simulink model "controller"  (R2024b)
settings: Solver=ode1  StartTime=0.0  StopTime=inf  FixedStep=0.01  RelTol=1e-3
libraries: robotlib x4, robotgazebolib x1
settings Model: Creator=abanesjo  LastModifiedBy=abanesjo

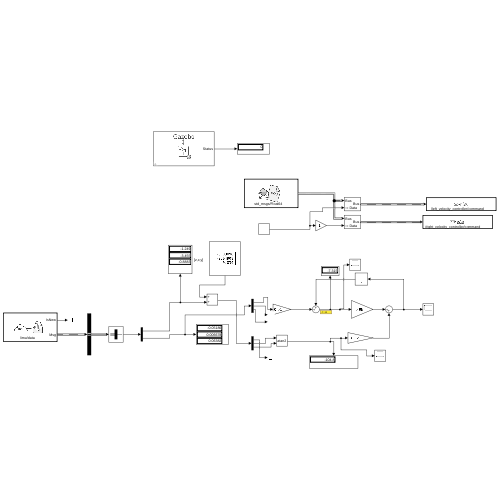
[thumbnail: Simulink's stored preview of the top-level diagram]
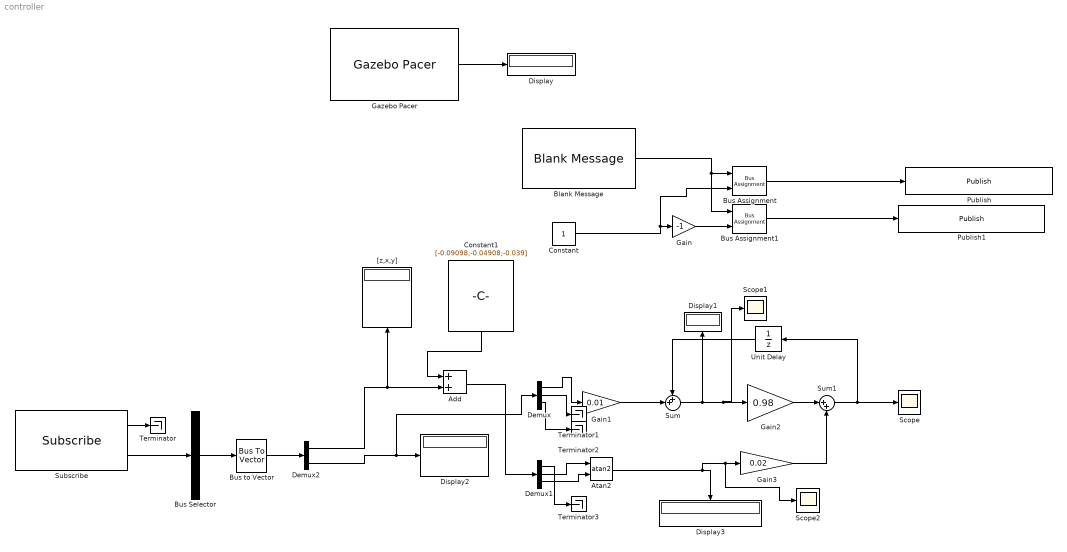
== system controller ==
  Add : Sum
  Atan2 : Trigonometry  Operator=atan2
  Blank Message : robotlib/Blank Message  messageClass=Message  entityType=std_msgs/Float64  messageType=std_msgs/Float64  SampleTime=inf  legacyBusStruct=off
  Bus Assignment : BusAssignment  AssignedSignals=Data
  Bus Assignment1 : BusAssignment  AssignedSignals=Data
  Bus Selector : BusSelector  OutputSignals=LinearAcceleration,AngularVelocity  OutputAsBus=on
  Bus to Vector : BusToVector
  Constant : Constant
  Constant1 : Constant  Value=[-0.09098;-0.04908;-0.039]  VectorParams1D=off
  Demux : Demux  Outputs=3
  Demux1 : Demux  Outputs=3
  Demux2 : Demux  Outputs=2
  Display{,1..3} (4 alike) : Display
  Gain : Gain  Gain=-1
  Gain1 : Gain  Gain=0.01
  Gain2 : Gain  Gain=0.98
  Gain3 : Gain  Gain=0.02
  Gazebo Pacer : robotgazebolib/Gazebo Pacer  ResetBehavior=Reset Gazebo simulation time and scene  SampleTime=0.01
  Publish : robotlib/Publish  topicSource=Specify your own  topic=/left_velocity_controller/command  messageType=std_msgs/Float64  legacyBusStruct=off  messageQueueLength=1
  Publish1 : robotlib/Publish  topicSource=Specify your own  topic=/right_velocity_controller/command  messageType=std_msgs/Float64  legacyBusStruct=off  messageQueueLength=1
  Scope : Scope
  Scope1 : Scope
  Scope2 : Scope
  Subscribe : robotlib/Subscribe  topicSource=Specify your own  topic=/imu/data  messageType=sensor_msgs/Imu  SampleTime=0.01  legacyBusStruct=off  messageQueueLength=1
  Sum : Sum  Inputs=++|
  Sum1 : Sum  Inputs=|++
  Terminator{,1..3} (4 alike) : Terminator
  Unit Delay : UnitDelay  SampleTime=-1  HasFrameUpgradeWarning=on
  "[z,x,y]" : Display
  wires:
  Bus Assignment/1 -> Publish/1
  Blank Message/1 -> Bus Assignment1/1, Bus Assignment/1
  Gazebo Pacer/1 -> Display/1
  Bus Assignment1/1 -> Publish1/1
  Gain/1 -> Bus Assignment1/2
  Constant/1 -> Bus Assignment/2, Gain/1
  Gain1/1 -> Sum/2
  Demux1/2 -> Atan2/1
  Demux1/1 -> Terminator3/1
  Demux/2 -> Terminator1/1
  Atan2/1 -> Scope2/1, Gain3/1, Display3/1
  Unit Delay/1 -> Sum/1
  Demux/1 -> Gain1/1
  Sum/1 -> Scope1/1, Gain2/1, Display1/1
  Sum1/1 -> Scope/1, Unit Delay/1
  Demux/3 -> Terminator2/1
  Constant1/1 -> Add/1
  Demux1/3 -> Atan2/2
  Gain3/1 -> Sum1/2
  Gain2/1 -> Sum1/1
  Add/1 -> Demux1/1
  Subscribe/1 -> Terminator/1
  Subscribe/2 -> Bus Selector/1
  Bus Selector/1 -> Bus to Vector/1
  Bus to Vector/1 -> Demux2/1
  Demux2/1 -> Add/2, "[z,x,y]"/1
  Demux2/2 -> Demux/1, Display2/1
